simulink model "simulacion_secuencia"  (R2023a)
settings: Solver=VariableStepAuto  StartTime=0.0  StopTime=4  RelTol=1e-3
values from neighbouring files (symbols this model uses):
  filtros = banco_decodificador(Fs, frecuencias_centrales, orden)    [main.m]    (also in sim_falla.m; sim_ideal.m; sim_real.m)
  Fs = 44000    [butter_digital_frec_resp.m]    (also in canal.m; main.m; sim_falla.m; sim_ideal.m)
libraries: dspstat3 x7, simulink x2
settings Model: Creator=leand  LastModifiedBy=lcampero

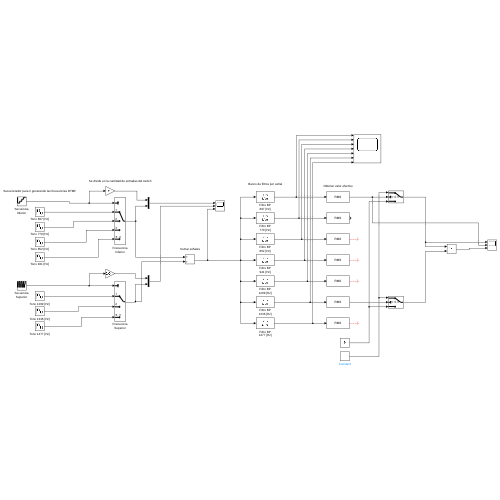
[thumbnail: Simulink's stored preview of the top-level diagram]
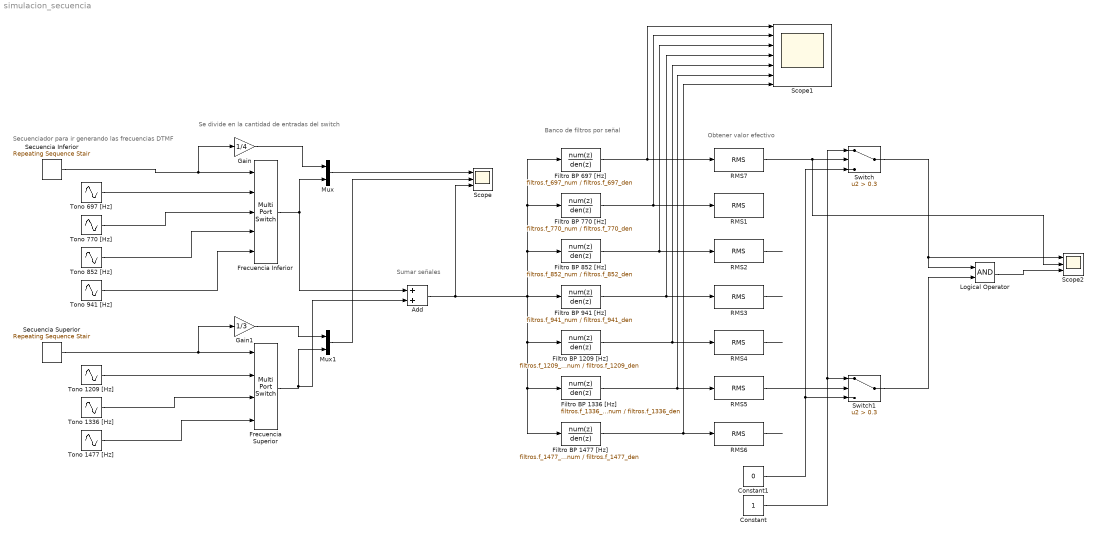
== system simulacion_secuencia ==
  note: Obtener valor efectivo
  note: Banco de filtros por señal
  note: Sumar señales
  note: Se divide en la cantidad de entradas del switch
  note: Secuenciador para ir generando las frecuencias DTMF
  Add : Sum
  Constant : Constant
  Constant1 : Constant  Value=0
  Filtro BP 1209 [Hz] : DiscreteTransferFcn  Numerator=filtros.f_1209_num  Denominator=filtros.f_1209_den  SampleTime=1/Fs
  Filtro BP 1336 [Hz] : DiscreteTransferFcn  Numerator=filtros.f_1336_num  Denominator=filtros.f_1336_den  SampleTime=1/Fs
  Filtro BP 1477 [Hz] : DiscreteTransferFcn  Numerator=filtros.f_1477_num  Denominator=filtros.f_1477_den  SampleTime=1/Fs
  Filtro BP 697 [Hz] : DiscreteTransferFcn  Numerator=filtros.f_697_num  Denominator=filtros.f_697_den  SampleTime=1/Fs
  Filtro BP 770 [Hz] : DiscreteTransferFcn  Numerator=filtros.f_770_num  Denominator=filtros.f_770_den  SampleTime=1/Fs
  Filtro BP 852 [Hz] : DiscreteTransferFcn  Numerator=filtros.f_852_num  Denominator=filtros.f_852_den  SampleTime=1/Fs
  Filtro BP 941 [Hz] : DiscreteTransferFcn  Numerator=filtros.f_941_num  Denominator=filtros.f_941_den  SampleTime=1/Fs
  Frecuencia Inferior : MultiPortSwitch  Inputs=4  SaturateOnIntegerOverflow=off  InputSameDT=off
  Frecuencia Superior : MultiPortSwitch  SaturateOnIntegerOverflow=off  InputSameDT=off
  Gain : Gain  Gain=1/4
  Gain1 : Gain  Gain=1/3
  Logical Operator : Logic  AllPortsSameDT=off  OutDataTypeStr=boolean
  Mux : Mux  Inputs=2
  Mux1 : Mux  Inputs=2
  RMS{1..7} (7 alike) : dspstat3/RMS  run=off  directionMode=Each column  dimension=1  InputProcessing=Columns as channels (frame based)  reset_popup=None
  Scope : Scope  NumInputPorts=3
  Scope1 : Scope  NumInputPorts=7
  Scope2 : Scope  NumInputPorts=3
  Secuencia Inferior : simulink/Sources/Repeating Sequence Stair  OutValues=[1 1 1 2 2 2 3 3 3 4 4 4].'  tsamp=1/4  OutMin=[]  OutMax=[]  OutDataTypeStr=double  OutputDataTypeScalingMode=double  OutDataType=fixdt(0,8)  ConRadixGroup=Best Precision: Vector-wise  OutScaling=2^-12
  Secuencia Superior : simulink/Sources/Repeating Sequence Stair  OutValues=[1 2 3 1 2 3 1 2 3 1 2 3].'  tsamp=1/4  OutMin=[]  OutMax=[]  OutDataTypeStr=double  OutputDataTypeScalingMode=double  OutDataType=fixdt(0,8)  ConRadixGroup=Best Precision: Vector-wise  OutScaling=2^-12
  Switch : Switch  Criteria=u2 > Threshold  Threshold=0.3  SaturateOnIntegerOverflow=off  InputSameDT=off
  Switch1 : Switch  Criteria=u2 > Threshold  Threshold=0.3  SaturateOnIntegerOverflow=off  InputSameDT=off
  Tono 1209 [Hz] : Sin  Frequency=2*pi*1209  SampleTime=1/Fs
  Tono 1336 [Hz] : Sin  Frequency=2*pi*1336  SampleTime=1/Fs
  Tono 1477 [Hz] : Sin  Frequency=2*pi*1477  SampleTime=1/Fs
  Tono 697 [Hz] : Sin  Frequency=2*pi*697  SampleTime=1/Fs
  Tono 770 [Hz] : Sin  Frequency=2*pi*770  SampleTime=1/Fs
  Tono 852 [Hz] : Sin  Frequency=2*pi*852  SampleTime=1/Fs
  Tono 941 [Hz] : Sin  Frequency=2*pi*941  SampleTime=1/Fs
  wires:
  Tono 1209 [Hz]/1 -> Frecuencia Superior/2
  Tono 1336 [Hz]/1 -> Frecuencia Superior/3
  Tono 1477 [Hz]/1 -> Frecuencia Superior/4
  Tono 697 [Hz]/1 -> Frecuencia Inferior/2
  Tono 770 [Hz]/1 -> Frecuencia Inferior/3
  Tono 852 [Hz]/1 -> Frecuencia Inferior/4
  Tono 941 [Hz]/1 -> Frecuencia Inferior/5
  Secuencia Inferior/1 -> Gain/1, Frecuencia Inferior/1
  Secuencia Superior/1 -> Frecuencia Superior/1, Gain1/1
  Frecuencia Inferior/1 -> Mux/2, Add/1
  Frecuencia Superior/1 -> Add/2, Mux1/2
  Mux/1 -> Scope/1
  Mux1/1 -> Scope/2
  Gain1/1 -> Mux1/1
  Gain/1 -> Mux/1
  Add/1 -> Scope/3, Filtro BP 852 [Hz]/1, Filtro BP 770 [Hz]/1, Filtro BP 697 [Hz]/1, Filtro BP 941 [Hz]/1, Filtro BP 1209 [Hz]/1, Filtro BP 1336 [Hz]/1, Filtro BP 1477 [Hz]/1
  Filtro BP 770 [Hz]/1 -> RMS1/1, Scope1/2
  Filtro BP 852 [Hz]/1 -> RMS2/1, Scope1/3
  Filtro BP 941 [Hz]/1 -> RMS3/1, Scope1/4
  Filtro BP 1209 [Hz]/1 -> RMS4/1, Scope1/5
  Filtro BP 1336 [Hz]/1 -> RMS5/1, Scope1/6
  Filtro BP 1477 [Hz]/1 -> RMS6/1, Scope1/7
  Filtro BP 697 [Hz]/1 -> RMS7/1, Scope1/1
  RMS2/1 -> ?
  RMS3/1 -> ?
  RMS4/1 -> ?
  RMS6/1 -> ?
  Constant/1 -> Switch/1, Switch1/1
  Constant1/1 -> Switch1/3, Switch/3
  RMS7/1 -> Scope2/2, Switch/2
  RMS5/1 -> Switch1/2
  Logical Operator/1 -> Scope2/3
  Switch1/1 -> Logical Operator/2
  Switch/1 -> Scope2/1, Logical Operator/1
